simulink model "dc_dc"  (R2018a)
settings: Solver=VariableStepDiscrete  StartTime=0.0  StopTime=0.01  RelTol=1e-3
libraries: powerlib x30, re_lib x2
settings Model: Creator=mwkane  LastModifiedBy=mwkane
settings SolverCC: AlgebraicLoopSolver=LineSearch

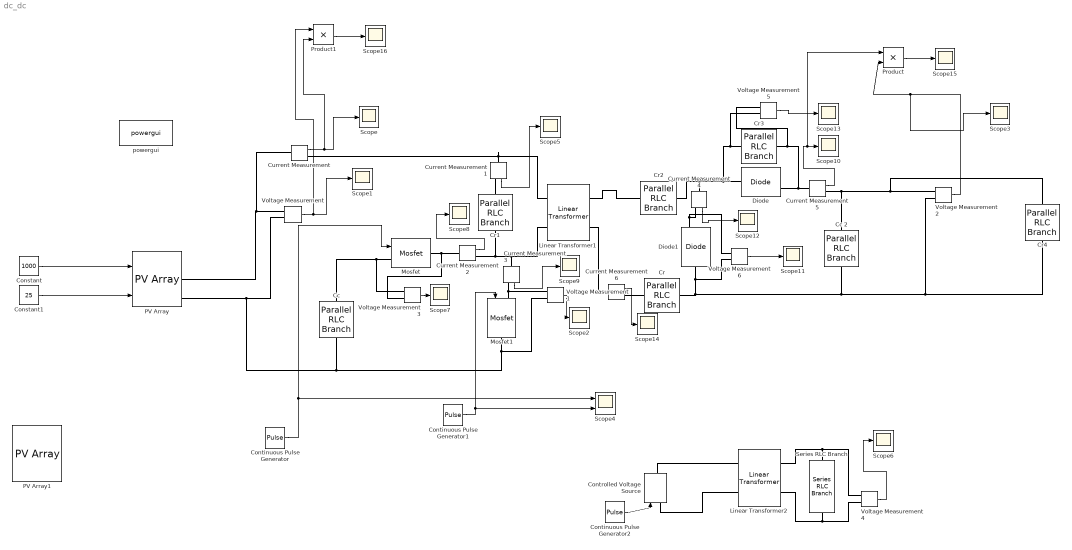
== system dc_dc ==
  "Cc " : powerlib/Elements/Parallel RLC Branch  LConnTagsString=a  RConnTagsString=__new0  BranchType=C  Resistance=1  Inductance=1e-3  SetiL0=off  InitialCurrent=0  Capacitance=2.2e-06  Setx0=off  InitialVoltage=0  Measurements=None
  Cc 2 : powerlib/Elements/Parallel RLC Branch  LConnTagsString=a  RConnTagsString=__new0  BranchType=C  Resistance=1  Inductance=1e-3  SetiL0=off  InitialCurrent=0  Capacitance=1e-6  Setx0=off  InitialVoltage=0  Measurements=None
  Constant : Constant  Value=1000
  Constant1 : Constant  Value=25
  Continuous Pulse Generator : DiscretePulseGenerator  PulseType=Time based  Amplitude=5  Period=0.00002  PulseWidth=40
  Continuous Pulse Generator1 : DiscretePulseGenerator  PulseType=Time based  Amplitude=5  Period=0.00002  PulseWidth=60  PhaseDelay=0.000008
  Continuous Pulse Generator2 : DiscretePulseGenerator  PulseType=Time based  Amplitude=24  Period=0.00002  PulseWidth=50
  Controlled Voltage Source : powerlib/Electrical Sources/Controlled Voltage Source  Initialize=on  Source_Type=AC  Amplitude=0  Phase=0  Frequency=0  Measurements=None
  Cr : powerlib/Elements/Parallel RLC Branch  LConnTagsString=a  RConnTagsString=__new0  BranchType=C  Resistance=1  Inductance=1e-3  SetiL0=off  InitialCurrent=0  Capacitance=2.4e-6  Setx0=off  InitialVoltage=0  Measurements=None
  Cr1 : powerlib/Elements/Parallel RLC Branch  LConnTagsString=a  RConnTagsString=__new0  BranchType=L  Resistance=1  Inductance=20e-6  SetiL0=off  InitialCurrent=0  Capacitance=2.4e-6  Setx0=off  InitialVoltage=0  Measurements=None
  Cr2 : powerlib/Elements/Parallel RLC Branch  LConnTagsString=a  RConnTagsString=__new0  BranchType=L  Resistance=1  Inductance=2.6e-6  SetiL0=off  InitialCurrent=0  Capacitance=2.4e-6  Setx0=off  InitialVoltage=0  Measurements=None
  Cr3 : powerlib/Elements/Parallel RLC Branch  LConnTagsString=a  RConnTagsString=__new0  BranchType=R  Resistance=1e6  Inductance=2.6e-6  SetiL0=off  InitialCurrent=0  Capacitance=2.4e-6  Setx0=off  InitialVoltage=0  Measurements=None
  Cr4 : powerlib/Elements/Parallel RLC Branch  LConnTagsString=a  RConnTagsString=__new0  BranchType=R  Resistance=1e3  Inductance=2.6e-6  SetiL0=off  InitialCurrent=0  Capacitance=2.4e-6  Setx0=off  InitialVoltage=0  Measurements=None
  Current Measurement{,1..6} (7 alike) : powerlib/Measurements/Current Measurement  PhasorSimulation=off  OutputType=Complex  PSBequivalent=0
  Diode : powerlib/Power Electronics/Diode  Ron=1  Lon=0  Vf=0.8  IC=0  UseSnubber=0  Rs=inf  Cs=0  Measurements=on
  Diode1 : powerlib/Power Electronics/Diode  Ron=0.01  Lon=0  Vf=0.8  IC=0  UseSnubber=0  Rs=inf  Cs=0  Measurements=on
  Linear Transformer1 : powerlib/Elements/Linear Transformer  UNITS=SI  NominalPower=[ 25 100e3 ]  winding1=[9 0 0]  winding2=[38 0 0]  ThreeWindings=off  winding3=[3.15e+05 3.969e+07 6316.9]  RmLm=[1e6 0]  Measurements=Magnetization current  DataType=on
  Linear Transformer2 : powerlib/Elements/Linear Transformer  UNITS=SI  NominalPower=[ 25 100e3 ]  winding1=[24.06 0 0]  winding2=[170 0 0]  ThreeWindings=off  winding3=[3.15e+05 3.969e+07 6316.9]  RmLm=[inf inf]  Measurements=Magnetization current  DataType=on
  Mosfet : powerlib/Power Electronics/Mosfet  Ron=0.1  Lon=0  Rd=0.01  Vfd=0  IC=0  Rs=1e5  Cs=inf  Measurements=off
  Mosfet1 : powerlib/Power Electronics/Mosfet  Ron=0.1  Lon=0  Rd=0.01  Vfd=0  IC=0  Rs=1e6  Cs=inf  Measurements=off
  PV Array : re_lib/Solar/PV Array  Npar=1  Nser=2  PlotType=array @ 25 deg.C & specified irradiances  S_vec="[ 1000  500  100 ]"  Temp_C_vec="[ 45 25  ]"  ModuleName=User-defined  PlotWhenSelected=off  Pm=179.9805  Ncell=36  Voc=24.06  Isc=9.77  Vm=19.67  Im=9.15  beta_Voc_pc=-0.28  alpha_Isc_pc=+0.04  beta_Voc=-0.067368  alpha_Isc=0.003908  IL=9.8911  I0=1.3829e-11  nI=0.95443  Rsh=60.4787  Rs=0.18212  BAL=off  Tc=1e-6  Tfilter=5e-5
  PV Array1 : re_lib/Solar/PV Array  Npar=1  Nser=1  PlotType=array @ 25 deg.C & specified irradiances  S_vec="[ 1000  500  100 ]"  Temp_C_vec="[ 45 25  ]"  ModuleName=User-defined  PlotWhenSelected=off  Pm=179.9805  Ncell=36  Voc=24.06  Isc=9.77  Vm=19.67  Im=9.15  beta_Voc_pc=-0.28  alpha_Isc_pc=+0.04  beta_Voc=-0.067368  alpha_Isc=0.003908  IL=9.8911  I0=1.3829e-11  nI=0.95443  Rsh=60.4787  Rs=0.18212  BAL=off  Tc=1e-6  Tfilter=5e-5
  Product : Product
  Product1 : Product
  Scope{,1..3,5..16} (16 alike) : Scope
  Scope4 : Scope  NumInputPorts=2
  Series RLC Branch : powerlib/Elements/Series RLC Branch  LConnTagsString=__new0  RConnTagsString=__new0  BranchType=R  Resistance=100  Inductance=1e-3  SetiL0=off  InitialCurrent=0  Capacitance=1e-6  Setx0=off  InitialVoltage=0  Measurements=None
  Voltage Measurement{,1..6} (7 alike) : powerlib/Measurements/Voltage Measurement  PhasorSimulation=off  OutputType=Complex  PSBequivalent=0
  powergui : powerlib/powergui  Priority=1  SimulationMode=Discrete  SampleTime=50e-10  frequency=60  Iterations=50  frequencyindice=0  Pbase=100e6  ErrMax=1e-4  UnitsV=kV  UnitsW=MW  buscounter=0  FunctionMessages=off  echomessages=off  EnableUseOfTLC=off  CurrentSourceSwitches=off  DisableSnubberDevices=off  DisableRonSwitches=off  DisableVfSwitches=off  DisplayEquations=off  SolverType=Tustin/Backward Euler (TBE)  Interpol=off  ExternalGateDelay=off  methode=off  Ts=100  x0status=blocks  SPID=on  SwTol=0  HookPort=off  RestoreLinks=warning  ResistiveCurrentMeasurement=off  Frange=[0:2:500]  Ylog=off  Xlog=on  ShowGrid=off  save=off  variable=ZData  structure=0  ZoomFFT=off  StartTime=0.0  cycles=1  DisplayStyle=1  fundamental=60  FreqAxis=off  MaxFrequency=1000  frequencyindicesteady=1  RmsSteady=1  display=off
  wires:
  Constant/1 -> PV Array/1
  Constant1/1 -> PV Array/2
  Current Measurement/1 -> Product1/2, Scope/1
  Voltage Measurement/1 -> Product1/1, Scope1/1
  Voltage Measurement2/1 -> Product/2, Scope3/1
  Continuous Pulse Generator/1 -> Mosfet/1, Scope4/1
  Continuous Pulse Generator1/1 -> Mosfet1/1, Scope4/2
  Voltage Measurement4/1 -> Scope6/1
  Continuous Pulse Generator2/1 -> Controlled Voltage Source/1
  Current Measurement1/1 -> Scope5/1
  Voltage Measurement1/1 -> Scope2/1
  Voltage Measurement3/1 -> Scope7/1
  Current Measurement2/1 -> Scope8/1
  Current Measurement3/1 -> Scope9/1
  Voltage Measurement5/1 -> Scope13/1
  Current Measurement4/1 -> Scope12/1
  Voltage Measurement6/1 -> Scope11/1
  Current Measurement5/1 -> Product/1, Scope10/1
  Current Measurement6/1 -> Scope14/1
  Product/1 -> Scope15/1
  Product1/1 -> Scope16/1
  connections:
  Voltage Measurement/LConn1 -- Current Measurement/LConn1 -- PV Array/RConn1
  Cr/RConn1 -- Cr4/RConn1 -- Voltage Measurement2/LConn2 -- Cc 2/RConn1 -- Voltage Measurement6/LConn2 -- Diode1/LConn1
  Diode/LConn1 -- Cr3/LConn1 -- Voltage Measurement5/LConn2 -- Cr2/RConn1 -- Current Measurement4/LConn1
  Voltage Measurement2/LConn1 -- Cr4/LConn1 -- Current Measurement5/RConn1 -- Cc 2/LConn1
  Current Measurement/RConn1 -- Current Measurement1/LConn1 -- Linear Transformer1/LConn1
  Mosfet1/LConn1 -- Current Measurement3/RConn1 -- Voltage Measurement1/LConn1
  Controlled Voltage Source/RConn1 -- Linear Transformer2/LConn1
  Controlled Voltage Source/LConn1 -- Linear Transformer2/LConn2
  Linear Transformer2/RConn1 -- Voltage Measurement4/LConn1 -- Series RLC Branch/LConn1
  Series RLC Branch/RConn1 -- Voltage Measurement4/LConn2 -- Linear Transformer2/RConn2
  PV Array/RConn2 -- "Cc "/RConn1 -- Voltage Measurement1/LConn2 -- Mosfet1/RConn1 -- Voltage Measurement/LConn2
  Linear Transformer1/RConn1 -- Cr2/LConn1
  Mosfet/LConn1 -- Voltage Measurement3/LConn1 -- "Cc "/LConn1
  Current Measurement1/RConn1 -- Cr1/LConn1
  Mosfet/RConn1 -- Current Measurement2/LConn1 -- Voltage Measurement3/LConn2
  Cr1/RConn1 -- Current Measurement3/LConn1 -- Linear Transformer1/LConn2 -- Current Measurement2/RConn1
  Diode/RConn1 -- Cr3/RConn1 -- Voltage Measurement5/LConn1 -- Current Measurement5/LConn1
  Current Measurement4/RConn1 -- Voltage Measurement6/LConn1 -- Diode1/RConn1
  Current Measurement6/RConn1 -- Cr/LConn1
  Current Measurement6/LConn1 -- Linear Transformer1/RConn2
